simulink model "eha_model_w_kf"  (R2015b)
settings: Solver=VariableStepAuto  StartTime=0.0  StopTime=10.0  RelTol=1e-3
values from neighbouring files (symbols this model uses):
  A = [ 1 0.001 0; 0 1 0.001; -557.02 -28.616 0.9418]    [eha_w_kalman_filter.m]
  B = [0 0 557.02]'    [eha_w_kalman_filter.m]
  C = H    [eha_w_kalman_filter.m]
  K = place(A,B,poles)    [eha_w_kalman_filter.m]    (also in run_eha.m)
  Nbar = rscale(sys,K)    [eha_w_kalman_filter.m]    (also in run_eha.m)
  P0 = 10*Q    [eha_w_kalman_filter.m]
  x0 = [0 0 0]'    [eha_w_kalman_filter.m]
undefined symbols (not defined in the file or in its folder): gaussian
libraries: simulink x1
settings Model: Creator=mathi  LastModifiedBy=Nicholas

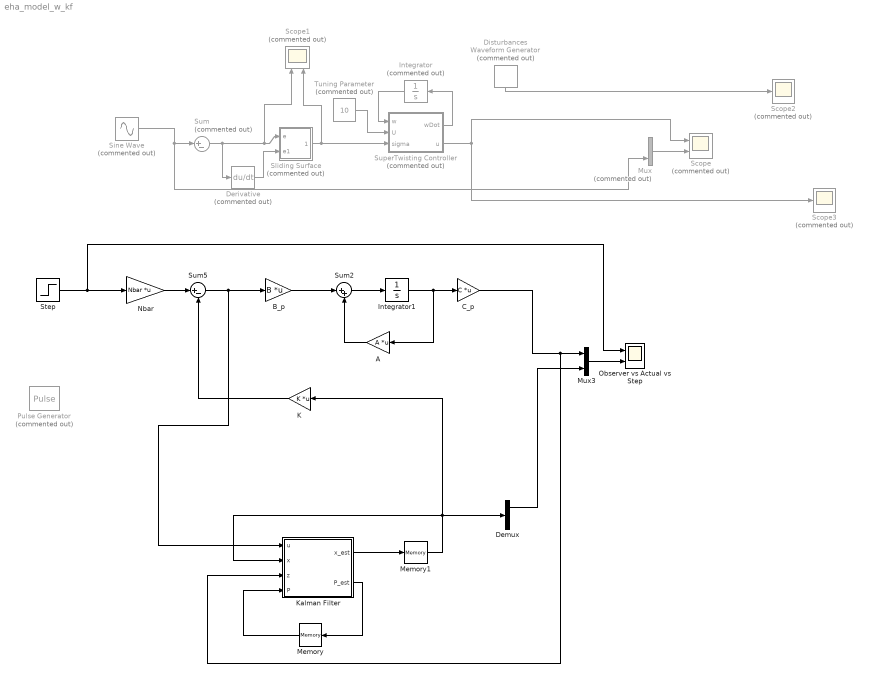
== system eha_model_w_kf ==
  A : Gain  Gain=A  Multiplication=Matrix(K*u)
  B_p : Gain  Gain=B  Multiplication=Matrix(K*u)
  C_p : Gain  Gain=C  Multiplication=Matrix(K*u)
  Demux : Demux  Outputs=3
  Derivative : Derivative  Commented=on
  Disturbances : simulink/Sources/Waveform Generator  Commented=on  OutMin=[]  OutMax=[]  OutDataTypeStr=double  SelectedSignal=1  Signals=gaussian(0,0,121313)  BlockNames=MultiportSwitch_d64598e6258c4fb  SampleTime=0.001
  Integrator : Integrator  Commented=on
  Integrator1 : Integrator  InitialCondition=x0
  K : Gain  Gain=K  Multiplication=Matrix(K*u)
  Kalman Filter : MATLAB Function  TreatAsAtomicUnit=on
  Memory : Memory  X0=P0
  Memory1 : Memory  X0=x0
  Mux : Mux  Commented=on  Inputs=2
  Mux3 : Mux  Inputs=2
  Nbar : Gain  Gain=Nbar  Multiplication=Matrix(K*u)
  "Observer vs Actual vs Step " : Scope  NumInputPorts=2
  Pulse Generator : DiscretePulseGenerator  Commented=on
  Scope : Scope  Commented=on  NumInputPorts=2
  Scope1 : Scope  Commented=on  NumInputPorts=2
  Scope2 : Scope  Commented=on
  Scope3 : Scope  Commented=on
  Sine Wave : Sin  Commented=on  Frequency=2  SampleTime=0
  "Sliding Surface " : Subsystem  Commented=on
  Step : Step  SampleTime=0
  Sum : Sum  Commented=on  Inputs=|+-
  Sum2 : Sum  Inputs=|++
  Sum5 : Sum  Inputs=|+-
  SuperTwisting Controller : MATLAB Function  Commented=on  TreatAsAtomicUnit=on
  Tuning Parameter : Constant  Commented=on  Value=10
  wires:
  Mux/1 -> Scope/2
  "Sliding Surface "/1(Sigma) -> SuperTwisting Controller/3(sigma), Scope1/2
  SuperTwisting Controller/1(wDot) -> Integrator/1
  Integrator/1 -> SuperTwisting Controller/1(w)
  Tuning Parameter/1 -> SuperTwisting Controller/2(U)
  Disturbances/1 -> Scope2/1
  Sum/1 -> "Sliding Surface "/1(e), Scope1/1, Derivative/1
  SuperTwisting Controller/2(u) -> Scope3/1, Scope/1
  Sine Wave/1 -> Sum/1, Mux/2
  Derivative/1 -> "Sliding Surface "/2(e1)
  Kalman Filter/2(P_est) -> Memory/1
  Kalman Filter/1(x_est) -> Memory1/1
  Memory/1 -> Kalman Filter/4(P)
  Memory1/1 -> Demux/1, K/1, Kalman Filter/2(x)
  A/1 -> Sum2/2
  Sum2/1 -> Integrator1/1
  Integrator1/1 -> A/1, C_p/1
  B_p/1 -> Sum2/1
  K/1 -> Sum5/2
  Sum5/1 -> Kalman Filter/1(u), B_p/1
  Step/1 -> "Observer vs Actual vs Step "/1, Nbar/1
  C_p/1 -> Kalman Filter/3(z), Mux3/1
  Nbar/1 -> Sum5/1
  Mux3/1 -> "Observer vs Actual vs Step "/2
  Demux/1 -> Mux3/2

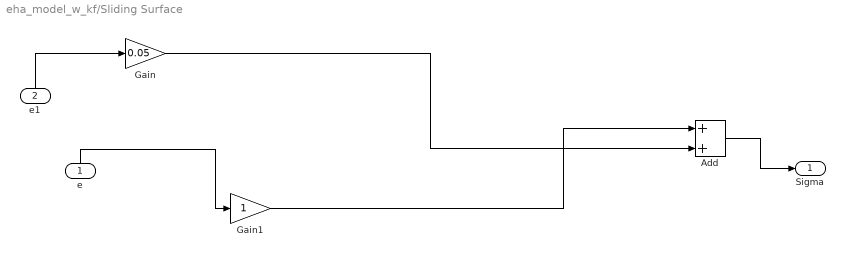
== system eha_model_w_kf/Sliding Surface  ==
  e : Inport
  e1 : Inport  Port=2
  Add : Sum
  Gain : Gain  Gain=0.05
  Gain1 : Gain
  Sigma : Outport
  wires:
  Add/1 -> Sigma/1
  e1/1 -> Gain/1
  Gain/1 -> Add/2
  e/1 -> Gain1/1
  Gain1/1 -> Add/1

== matlab function eha_model_w_kf/Kalman Filter ==
  data: u input; x_est output; x input; z input; P input; P_est output
function [x_est, P_est] = fcn(u,x,z,P)
%#codegen
Q = [ 1 0 0; 0 1 0; 0 0 100];
A = [ 1 0.001 0; 0 1 0.001; -557.02 -28.616 0.9418];
B = [0 0 557.02]';
H = [1 0 0];
R = 10;

x_next = A*x + B*u;
P_next = A * P * A' + Q;


% Compute Kalman gain factor:
K_f =P*H'*pinv(H*P*H'+ R);
% Correction based on observation:
x_est = x_next + K_f*(z-H*x_next);
P_est = P_next - K_f*H*P_next;

== matlab function eha_model_w_kf/SuperTwisting Controller ==
  data: w input; U input; wDot output; u output; sigma input
function [wDot,u] = fcn(w,U,sigma)

lambda = sqrt(U);
W = 1.1*U;

u = lambda*sqrt(abs(sigma))*sign(sigma) + w;
 wDot = W*sign(sigma);
